simulink model "finite_diff"  (R2019a)
settings: Solver=VariableStepAuto  StartTime=0.0  StopTime=1  RelTol=1e-3
values from neighbouring files (symbols this model uses):
  x_dot = [c_s_n_dot; c_s_p_dot; c_e_dot; T1_dot; T2_dot; delta_sei_dot]    [ode_spmet_cccv.m]    (also in x_dot.mat = [6.01011616268e-17 1.82143271062e-15 -1.75993084831e-15 -4.4)
undefined symbols (not defined in the file or in its folder): x0_nom
settings Model: Creator=ztakeo  LastModifiedBy=ztakeo

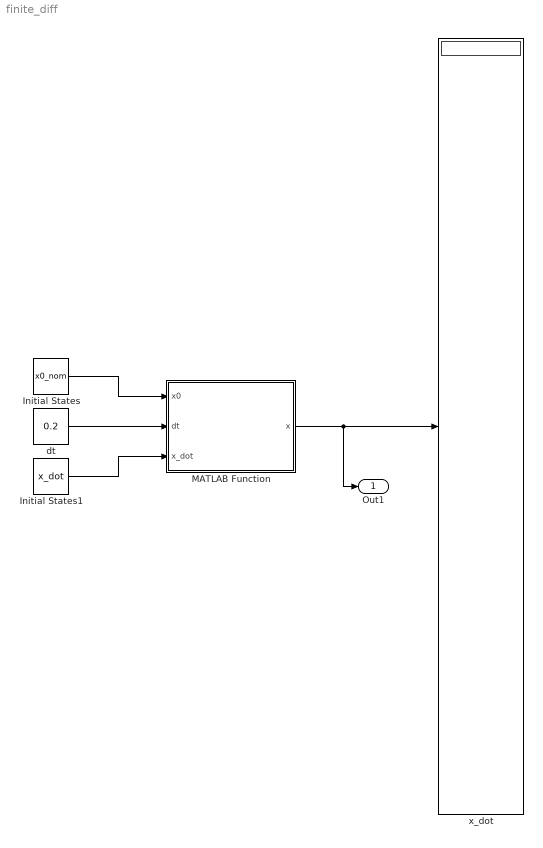
== system finite_diff ==
  Initial States : Constant  Value=x0_nom
  Initial States1 : Constant  Value=x_dot
  MATLAB Function : MATLAB Function  TreatAsAtomicUnit=on
  dt : Constant  Value=0.2
  x_dot : Display
  Out1 : Outport
  wires:
  Initial States/1 -> MATLAB Function/1(x0)
  dt/1 -> MATLAB Function/2(dt)
  Initial States1/1 -> MATLAB Function/3(x_dot)
  MATLAB Function/1(x) -> Out1/1, x_dot/1

== matlab function finite_diff/MATLAB Function ==
  data: x0 input; x output; dt input; x_dot input
%% Simple function for stepping forward based on finite difference scheme
function x = fcn(x0,dt,x_dot)
    x = x0 + dt*x_dot;
end
